simulink model "neighbour_and_local"  (R2020a)
settings: Solver=ode15s  StartTime=0.0  StopTime=200  FixedStep=1e-3
values from neighbouring files (symbols this model uses):
  A = A-B*Kctrl    [project2.m]
  Adj = tril(ones(6),-1) - tril(ones(6),-2)    [project2.m]
  B = [0; -9.9453]    [project2.m]
  c = ctemp*10    [project2.m]
  C = [708.27 0]    [project2.m]
  D = 0    [project2.m]
  Fl = -Fn    [project2.m]
  Fn = Pn*C'*inv(R)    [project2.m]
  K = inv(R)*B'*Pk    [project2.m]
  Pinning = zeros(6)    [project2.m]
  x0 = [0,0]    [project2.m]
  x1 = [0;1/707.27]    [project2.m]
settings Model: Creator=fmare  LastModifiedBy=fmare

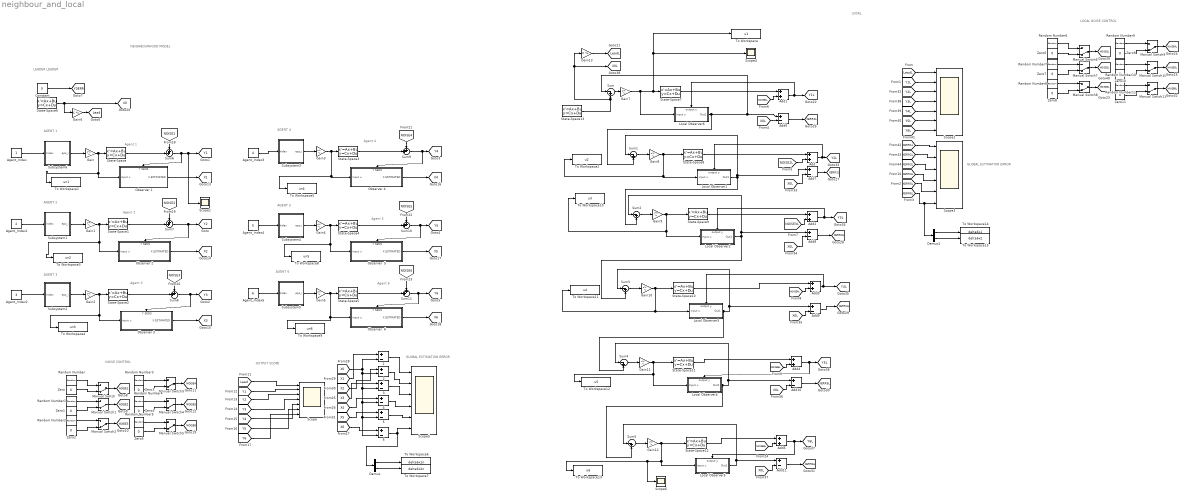
== system neighbour_and_local ==
  note: GLOBAL ESTIMATION ERROR
  note: AGENT 2
  note: NEIGHBOURHOOD MODEL
  note: OUTPUT SCOPE
  note: NOISE CONTROL
  note: Agent 6
  note: Agent 5
  note: Agent 4
  note: Agent 3
  note: Agent 1
  note: Agent 2
  note: AGENT 3
  note: AGENT 4
  note: AGENT 5
  note: AGENT 6
  note: AGENT 1
  note: LEADER
      | LEADER
  note: LOCAL NOISE CONTROL
  note: LOCAL
  note: GLOBAL ESTIMATION ERROR
  {1..6} (6 alike) : Sum  Inputs=+-
  Add{,1..5} (6 alike) : Sum
  Add{6..11} (6 alike) : Sum  Inputs=+-
  Agent_Index : Constant
  Agent_Index1 : Constant  Value=2
  Agent_Index2 : Constant  Value=3
  Agent_Index3 : Constant  Value=4
  Agent_Index4 : Constant  Value=5
  Agent_Index5 : Constant  Value=6
  Constant : Constant  Value=0
  Demux : Demux  Outputs=2
  Demux1 : Demux  Outputs=2
  Gain{,1..5,7..12} (12 alike) : Gain  Gain=c*K  Multiplication=Matrix(K*u)
  Gain13 : Gain  Gain=C  Multiplication=Matrix(K*u)
  Gain6 : Gain  Gain=C  Multiplication=Matrix(K*u)
  Local Observer1 : Subsystem
      settings: PortSchema="{\"entries\":[{\"content\":{\"sides\":[{\"content\":{\"connectorIds\":[\"In1\"]},\"type\":\"ConnectorPlacement.EquallySpacedRectSide\",\"uuid\":\"ce67de7f-91c0-4754-b336-8169ed1c06a3\"},{\"content\":{\"connectorIds\":[\"Out1\"],\"side\":\"RIGHT\"},\"type\":\"ConnectorPlacement.EquallySpacedRectSide\",\"uuid\":\"6e6b0d4a-9d22-40e2-b393-8f2d03ad4e6d\"},{\"content\":{\"connectorIds\":[\"In2\"],\"side\":\"TOP\"},\"type\":\"ConnectorPlacement.EquallySpacedRectSide\",\"uuid\":\"826e64ba-5ab3-47cb-8ff5-a35c256fda47\"}]},\"type\":\"ConnectorPlacement.EquallySpacedConnector\",\"uuid\":\"cb3a4a79-4d46-4198-893f-ba43cc9ed20a\"}],\"packageUris\":[\"http://schema.mathworks.com/mf0/Connector/19700101\"],\"version\":\"1.0\"}"
  Local Observer2 : Subsystem
      settings: ErrorFcn=x0(:,3)  PortSchema="{\"entries\":[{\"content\":{\"sides\":[{\"content\":{\"connectorIds\":[\"In1\"]},\"type\":\"ConnectorPlacement.EquallySpacedRectSide\",\"uuid\":\"ce67de7f-91c0-4754-b336-8169ed1c06a3\"},{\"content\":{\"connectorIds\":[\"Out1\"],\"side\":\"RIGHT\"},\"type\":\"ConnectorPlacement.EquallySpacedRectSide\",\"uuid\":\"6e6b0d4a-9d22-40e2-b393-8f2d03ad4e6d\"},{\"content\":{\"connectorIds\":[\"In2\"],\"side\":\"TOP\"},\"type\":\"ConnectorPlacement.EquallySpacedRectSide\",\"uuid\":\"826e64ba-5ab3-47cb-8ff5-a35c256fda47\"}]},\"type\":\"ConnectorPlacement.EquallySpacedConnector\",\"uuid\":\"cb3a4a79-4d46-4198-893f-ba43cc9ed20a\"}],\"packageUris\":[\"http://schema.mathworks.com/mf0/Connector/19700101\"],\"version\":\"1.0\"}"
  Local Observer3 : Subsystem
      settings: PortSchema="{\"entries\":[{\"content\":{\"sides\":[{\"content\":{\"connectorIds\":[\"In1\"]},\"type\":\"ConnectorPlacement.EquallySpacedRectSide\",\"uuid\":\"ce67de7f-91c0-4754-b336-8169ed1c06a3\"},{\"content\":{\"connectorIds\":[\"Out1\"],\"side\":\"RIGHT\"},\"type\":\"ConnectorPlacement.EquallySpacedRectSide\",\"uuid\":\"6e6b0d4a-9d22-40e2-b393-8f2d03ad4e6d\"},{\"content\":{\"connectorIds\":[\"In2\"],\"side\":\"TOP\"},\"type\":\"ConnectorPlacement.EquallySpacedRectSide\",\"uuid\":\"826e64ba-5ab3-47cb-8ff5-a35c256fda47\"}]},\"type\":\"ConnectorPlacement.EquallySpacedConnector\",\"uuid\":\"cb3a4a79-4d46-4198-893f-ba43cc9ed20a\"}],\"packageUris\":[\"http://schema.mathworks.com/mf0/Connector/19700101\"],\"version\":\"1.0\"}"
  Local Observer4 : Subsystem
      settings: PortSchema="{\"entries\":[{\"content\":{\"sides\":[{\"content\":{\"connectorIds\":[\"In1\"]},\"type\":\"ConnectorPlacement.EquallySpacedRectSide\",\"uuid\":\"ce67de7f-91c0-4754-b336-8169ed1c06a3\"},{\"content\":{\"connectorIds\":[\"Out1\"],\"side\":\"RIGHT\"},\"type\":\"ConnectorPlacement.EquallySpacedRectSide\",\"uuid\":\"6e6b0d4a-9d22-40e2-b393-8f2d03ad4e6d\"},{\"content\":{\"connectorIds\":[\"In2\"],\"side\":\"TOP\"},\"type\":\"ConnectorPlacement.EquallySpacedRectSide\",\"uuid\":\"826e64ba-5ab3-47cb-8ff5-a35c256fda47\"}]},\"type\":\"ConnectorPlacement.EquallySpacedConnector\",\"uuid\":\"cb3a4a79-4d46-4198-893f-ba43cc9ed20a\"}],\"packageUris\":[\"http://schema.mathworks.com/mf0/Connector/19700101\"],\"version\":\"1.0\"}"
  Local Observer5 : Subsystem
      settings: PortSchema="{\"entries\":[{\"content\":{\"sides\":[{\"content\":{\"connectorIds\":[\"In1\"]},\"type\":\"ConnectorPlacement.EquallySpacedRectSide\",\"uuid\":\"ce67de7f-91c0-4754-b336-8169ed1c06a3\"},{\"content\":{\"connectorIds\":[\"Out1\"],\"side\":\"RIGHT\"},\"type\":\"ConnectorPlacement.EquallySpacedRectSide\",\"uuid\":\"6e6b0d4a-9d22-40e2-b393-8f2d03ad4e6d\"},{\"content\":{\"connectorIds\":[\"In2\"],\"side\":\"TOP\"},\"type\":\"ConnectorPlacement.EquallySpacedRectSide\",\"uuid\":\"826e64ba-5ab3-47cb-8ff5-a35c256fda47\"}]},\"type\":\"ConnectorPlacement.EquallySpacedConnector\",\"uuid\":\"cb3a4a79-4d46-4198-893f-ba43cc9ed20a\"}],\"packageUris\":[\"http://schema.mathworks.com/mf0/Connector/19700101\"],\"version\":\"1.0\"}"
  Local Observer6 : Subsystem
      settings: PortSchema="{\"entries\":[{\"content\":{\"sides\":[{\"content\":{\"connectorIds\":[\"In1\"]},\"type\":\"ConnectorPlacement.EquallySpacedRectSide\",\"uuid\":\"ce67de7f-91c0-4754-b336-8169ed1c06a3\"},{\"content\":{\"connectorIds\":[\"Out1\"],\"side\":\"RIGHT\"},\"type\":\"ConnectorPlacement.EquallySpacedRectSide\",\"uuid\":\"6e6b0d4a-9d22-40e2-b393-8f2d03ad4e6d\"},{\"content\":{\"connectorIds\":[\"In2\"],\"side\":\"TOP\"},\"type\":\"ConnectorPlacement.EquallySpacedRectSide\",\"uuid\":\"826e64ba-5ab3-47cb-8ff5-a35c256fda47\"}]},\"type\":\"ConnectorPlacement.EquallySpacedConnector\",\"uuid\":\"cb3a4a79-4d46-4198-893f-ba43cc9ed20a\"}],\"packageUris\":[\"http://schema.mathworks.com/mf0/Connector/19700101\"],\"version\":\"1.0\"}"
  Manual Switch{,1..11} (12 alike) : ManualSwitch  CurrentSetting=0
  Observer  5 : Subsystem
      settings: PortSchema="{\"entries\":[{\"content\":{\"sides\":[{\"content\":{\"connectorIds\":[\"In1\"]},\"type\":\"ConnectorPlacement.EquallySpacedRectSide\",\"uuid\":\"b93c2c7e-291f-4b9d-8fda-1b2b099801ba\"},{\"content\":{\"connectorIds\":[\"Out1\"],\"side\":\"RIGHT\"},\"type\":\"ConnectorPlacement.EquallySpacedRectSide\",\"uuid\":\"bce36e82-6a20-4166-b86c-027f3aa24e2d\"},{\"content\":{\"connectorIds\":[\"In2\"],\"side\":\"TOP\"},\"type\":\"ConnectorPlacement.EquallySpacedRectSide\",\"uuid\":\"6cc367c2-dbc2-4b10-a825-48e36dcd66f7\"}]},\"type\":\"ConnectorPlacement.EquallySpacedConnector\",\"uuid\":\"fae6adff-b2a2-4da1-a9d8-7a0ab3ce0116\"}],\"packageUris\":[\"http://schema.mathworks.com/mf0/Connector/R2020b\"],\"version\":\"1.0\"}"
  Observer  6 : Subsystem
      settings: PortSchema="{\"entries\":[{\"content\":{\"sides\":[{\"content\":{\"connectorIds\":[\"In1\"]},\"type\":\"ConnectorPlacement.EquallySpacedRectSide\",\"uuid\":\"b93c2c7e-291f-4b9d-8fda-1b2b099801ba\"},{\"content\":{\"connectorIds\":[\"Out1\"],\"side\":\"RIGHT\"},\"type\":\"ConnectorPlacement.EquallySpacedRectSide\",\"uuid\":\"bce36e82-6a20-4166-b86c-027f3aa24e2d\"},{\"content\":{\"connectorIds\":[\"In2\"],\"side\":\"TOP\"},\"type\":\"ConnectorPlacement.EquallySpacedRectSide\",\"uuid\":\"6cc367c2-dbc2-4b10-a825-48e36dcd66f7\"}]},\"type\":\"ConnectorPlacement.EquallySpacedConnector\",\"uuid\":\"fae6adff-b2a2-4da1-a9d8-7a0ab3ce0116\"}],\"packageUris\":[\"http://schema.mathworks.com/mf0/Connector/R2020b\"],\"version\":\"1.0\"}"
  Observer 1 : Subsystem
      settings: PortSchema="{\"entries\":[{\"content\":{\"sides\":[{\"content\":{\"connectorIds\":[\"In1\"]},\"type\":\"ConnectorPlacement.EquallySpacedRectSide\",\"uuid\":\"b93c2c7e-291f-4b9d-8fda-1b2b099801ba\"},{\"content\":{\"connectorIds\":[\"Out1\"],\"side\":\"RIGHT\"},\"type\":\"ConnectorPlacement.EquallySpacedRectSide\",\"uuid\":\"bce36e82-6a20-4166-b86c-027f3aa24e2d\"},{\"content\":{\"connectorIds\":[\"In2\"],\"side\":\"TOP\"},\"type\":\"ConnectorPlacement.EquallySpacedRectSide\",\"uuid\":\"6cc367c2-dbc2-4b10-a825-48e36dcd66f7\"}]},\"type\":\"ConnectorPlacement.EquallySpacedConnector\",\"uuid\":\"fae6adff-b2a2-4da1-a9d8-7a0ab3ce0116\"}],\"packageUris\":[\"http://schema.mathworks.com/mf0/Connector/R2020b\"],\"version\":\"1.0\"}"
  Observer 2 : Subsystem
      settings: PortSchema="{\"entries\":[{\"content\":{\"sides\":[{\"content\":{\"connectorIds\":[\"In1\"]},\"type\":\"ConnectorPlacement.EquallySpacedRectSide\",\"uuid\":\"b93c2c7e-291f-4b9d-8fda-1b2b099801ba\"},{\"content\":{\"connectorIds\":[\"Out1\"],\"side\":\"RIGHT\"},\"type\":\"ConnectorPlacement.EquallySpacedRectSide\",\"uuid\":\"bce36e82-6a20-4166-b86c-027f3aa24e2d\"},{\"content\":{\"connectorIds\":[\"In2\"],\"side\":\"TOP\"},\"type\":\"ConnectorPlacement.EquallySpacedRectSide\",\"uuid\":\"6cc367c2-dbc2-4b10-a825-48e36dcd66f7\"}]},\"type\":\"ConnectorPlacement.EquallySpacedConnector\",\"uuid\":\"fae6adff-b2a2-4da1-a9d8-7a0ab3ce0116\"}],\"packageUris\":[\"http://schema.mathworks.com/mf0/Connector/R2020b\"],\"version\":\"1.0\"}"
  Observer 3 : Subsystem
      settings: PortSchema="{\"entries\":[{\"content\":{\"sides\":[{\"content\":{\"connectorIds\":[\"In1\"]},\"type\":\"ConnectorPlacement.EquallySpacedRectSide\",\"uuid\":\"b93c2c7e-291f-4b9d-8fda-1b2b099801ba\"},{\"content\":{\"connectorIds\":[\"Out1\"],\"side\":\"RIGHT\"},\"type\":\"ConnectorPlacement.EquallySpacedRectSide\",\"uuid\":\"bce36e82-6a20-4166-b86c-027f3aa24e2d\"},{\"content\":{\"connectorIds\":[\"In2\"],\"side\":\"TOP\"},\"type\":\"ConnectorPlacement.EquallySpacedRectSide\",\"uuid\":\"6cc367c2-dbc2-4b10-a825-48e36dcd66f7\"}]},\"type\":\"ConnectorPlacement.EquallySpacedConnector\",\"uuid\":\"fae6adff-b2a2-4da1-a9d8-7a0ab3ce0116\"}],\"packageUris\":[\"http://schema.mathworks.com/mf0/Connector/R2020b\"],\"version\":\"1.0\"}"
  Observer 4 : Subsystem
      settings: PortSchema="{\"entries\":[{\"content\":{\"sides\":[{\"content\":{\"connectorIds\":[\"In1\"]},\"type\":\"ConnectorPlacement.EquallySpacedRectSide\",\"uuid\":\"b93c2c7e-291f-4b9d-8fda-1b2b099801ba\"},{\"content\":{\"connectorIds\":[\"Out1\"],\"side\":\"RIGHT\"},\"type\":\"ConnectorPlacement.EquallySpacedRectSide\",\"uuid\":\"bce36e82-6a20-4166-b86c-027f3aa24e2d\"},{\"content\":{\"connectorIds\":[\"In2\"],\"side\":\"TOP\"},\"type\":\"ConnectorPlacement.EquallySpacedRectSide\",\"uuid\":\"6cc367c2-dbc2-4b10-a825-48e36dcd66f7\"}]},\"type\":\"ConnectorPlacement.EquallySpacedConnector\",\"uuid\":\"fae6adff-b2a2-4da1-a9d8-7a0ab3ce0116\"}],\"packageUris\":[\"http://schema.mathworks.com/mf0/Connector/R2020b\"],\"version\":\"1.0\"}"
  Random Number{,1..5} (6 alike) : RandomNumber  Variance=0.5  SampleTime=0.1
  Random Number{6..11} (6 alike) : RandomNumber  SampleTime=0.1
  Scope : Scope  NumInputPorts=7
  Scope1 : Scope
  Scope2 : Scope  NumInputPorts=7
  Scope3 : Scope  NumInputPorts=6
  Scope4 : Scope
  Scope5 : Scope  NumInputPorts=6
  Scope6 : Scope
  State-Space : StateSpace  A=A  B=B  C=C  D=D  InitialCondition=x0(:,1)
  State-Space1 : StateSpace  A=A  B=B  C=C  D=D  InitialCondition=x0(:,2)
  State-Space10 : StateSpace  A=A  B=B  C=C  D=D  InitialCondition=x0(:,4)
  State-Space11 : StateSpace  A=A  B=B  C=C  D=D  InitialCondition=x0(:,5)
  State-Space12 : StateSpace  A=A  B=B  C=C  D=D  InitialCondition=x0(:,6)
  State-Space13 : StateSpace  A=A  B=B  C=eye(2)  D=zeros(2,1)  InitialCondition=x1
  State-Space2 : StateSpace  A=A  B=B  C=C  D=D  InitialCondition=x0(:,3)
  State-Space3 : StateSpace  A=A  B=B  C=C  D=D  InitialCondition=x0(:,4)
  State-Space4 : StateSpace  A=A  B=B  C=C  D=D  InitialCondition=x0(:,5)
  State-Space5 : StateSpace  A=A  B=B  C=C  D=D  InitialCondition=x0(:,6)
  State-Space6 : StateSpace  A=A  B=B  C=eye(2)  D=zeros(2,1)  InitialCondition=x1
  State-Space7 : StateSpace  A=A  B=B  C=C  D=D  InitialCondition=x0(:,1)
  State-Space8 : StateSpace  A=A  B=B  C=C  D=D  InitialCondition=x0(:,2)
  State-Space9 : StateSpace  A=A  B=B  C=C  D=D  InitialCondition=x0(:,3)
  Subsystem1 : Subsystem
  Subsystem2 : Subsystem
  Subsystem3 : Subsystem
  Subsystem4 : Subsystem
  Subsystem5 : Subsystem
  Subsystem6 : Subsystem
  Sum{,1..5} (6 alike) : Sum  Inputs=|-+
  Sum{6..11} (6 alike) : Sum  Inputs=++|
  To Workspace : ToWorkspace  VariableName=u1  SaveFormat=Timeseries  SampleTime=-1
      settings: Save2DSignal=2-D array (concatenate along first dimension)
  To Workspace1 : ToWorkspace  VariableName=un1  SaveFormat=Timeseries  SampleTime=-1
      settings: Save2DSignal=2-D array (concatenate along first dimension)
  To Workspace10 : ToWorkspace  VariableName=u3  SaveFormat=Timeseries  SampleTime=-1
      settings: Save2DSignal=2-D array (concatenate along first dimension)
  To Workspace11 : ToWorkspace  VariableName=u4  SaveFormat=Timeseries  SampleTime=-1
      settings: Save2DSignal=2-D array (concatenate along first dimension)
  To Workspace12 : ToWorkspace  VariableName=u5  SaveFormat=Timeseries  SampleTime=-1
      settings: Save2DSignal=2-D array (concatenate along first dimension)
  To Workspace13 : ToWorkspace  VariableName=u6  SaveFormat=Timeseries  SampleTime=-1
      settings: Save2DSignal=2-D array (concatenate along first dimension)
  To Workspace14 : ToWorkspace  VariableName=delta6x1  SaveFormat=Timeseries  SampleTime=-1
      settings: Save2DSignal=2-D array (concatenate along first dimension)
  To Workspace15 : ToWorkspace  VariableName=delta6x2  SaveFormat=Timeseries  SampleTime=-1
      settings: Save2DSignal=2-D array (concatenate along first dimension)
  To Workspace2 : ToWorkspace  VariableName=u2  SaveFormat=Timeseries  SampleTime=-1
      settings: Save2DSignal=2-D array (concatenate along first dimension)
  To Workspace3 : ToWorkspace  VariableName=un2  SaveFormat=Timeseries  SampleTime=-1
      settings: Save2DSignal=2-D array (concatenate along first dimension)
  To Workspace4 : ToWorkspace  VariableName=un3  SaveFormat=Timeseries  SampleTime=-1
      settings: Save2DSignal=2-D array (concatenate along first dimension)
  To Workspace5 : ToWorkspace  VariableName=un4  SaveFormat=Timeseries  SampleTime=-1
      settings: Save2DSignal=2-D array (concatenate along first dimension)
  To Workspace6 : ToWorkspace  VariableName=delta6x1n  SaveFormat=Timeseries  SampleTime=-1
      settings: Save2DSignal=2-D array (concatenate along first dimension)
  To Workspace7 : ToWorkspace  VariableName=delta6x2n  SaveFormat=Timeseries  SampleTime=-1
      settings: Save2DSignal=2-D array (concatenate along first dimension)
  To Workspace8 : ToWorkspace  VariableName=un5  SaveFormat=Timeseries  SampleTime=-1
      settings: Save2DSignal=2-D array (concatenate along first dimension)
  To Workspace9 : ToWorkspace  VariableName=un6  SaveFormat=Timeseries  SampleTime=-1
      settings: Save2DSignal=2-D array (concatenate along first dimension)
  Zero{,1..11} (12 alike) : Constant  Value=0  OutDataTypeStr=Inherit: Inherit via back propagation
  tag scope: Lead=global, LeadL=global, NOISE1=global, NOISE1L=global, NOISE2=global, NOISE2L=global, NOISE3=global, NOISE3L=global, NOISE4=global, NOISE4L=global, NOISE5=global, NOISE5L=global, NOISE6=global, NOISE6L=global, X0=global, X0L=global, X1=global, X2=global, X3=global, X4=global, X5=global, X6=global, XERR1L=global, XERR2L=global, XERR3L=global, XERR4L=global, XERR5L=global, XERR6L=global, Y0ERR=global, Y1=global, Y1L=global, Y2=global, Y2L=global, Y3=global, Y3L=global, Y4=global, Y4L=global, Y5=global, Y5L=global, Y6=global, Y6L=global
  wires:
  State-Space3/1 -> Sum9/2
  State-Space4/1 -> Sum10/2
  State-Space6/1 -> [X0], Gain6/1
  State-Space5/1 -> Sum11/2
  State-Space/1 -> Sum6/2
  Gain2/1 -> To Workspace4/1, Observer 3/1(input u), State-Space2/1
  Gain1/1 -> To Workspace3/1, Observer 2/1(input u), State-Space1/1
  Gain5/1 -> State-Space5/1, To Workspace9/1, Observer  6/1(input u)
  State-Space2/1 -> Sum8/2
  Gain/1 -> To Workspace1/1, Observer 1/1(input u), State-Space/1
  State-Space1/1 -> Sum7/2
  Gain3/1 -> State-Space3/1, To Workspace5/1, Observer 4/1(input u)
  Observer 1/1(X ESTIMATED) -> [X1]
  Observer 2/1(X ESTIMATED) -> [X2]
  Observer 3/1(X ESTIMATED) -> [X3]
  Observer 4/1(X ESTIMATED) -> [X4]
  Observer  5/1(X ESTIMATED) -> [X5]
  Observer  6/1(X ESTIMATED) -> [X6]
  [Lead] -> Scope/1
  [Y1] -> Scope/2
  [Y2] -> Scope/3
  [Y3] -> Scope/4
  [Y4] -> Scope/5
  [Y5] -> Scope/6
  [Y6] -> Scope/7
  Gain6/1 -> [Lead]
  Constant/1 -> [Y0ERR]
  Sum6/1 -> Scope1/1, [Y1], Observer 1/2(Y SENS)
  Sum10/1 -> [Y5], Observer  5/2(Y SENS)
  Sum9/1 -> [Y4], Observer 4/2(Y SENS)
  Sum8/1 -> [Y3], Observer 3/2(Y SENS)
  Sum7/1 -> [Y2], Observer 2/2(Y SENS)
  [NOISE2] -> Sum7/1
  [NOISE1] -> Sum6/1
  [NOISE3] -> Sum8/1
  [NOISE4] -> Sum9/1
  [NOISE5] -> Sum10/1
  [NOISE6] -> Sum11/1
  Manual Switch/1 -> [NOISE1]
  Random Number/1 -> Manual Switch/1
  Zero/1 -> Manual Switch/2
  Random Number1/1 -> Manual Switch1/1
  Manual Switch1/1 -> [NOISE2]
  Zero1/1 -> Manual Switch1/2
  Random Number2/1 -> Manual Switch2/1
  Manual Switch2/1 -> [NOISE3]
  Zero2/1 -> Manual Switch2/2
  Random Number3/1 -> Manual Switch3/1
  Manual Switch3/1 -> [NOISE4]
  Zero3/1 -> Manual Switch3/2
  Random Number4/1 -> Manual Switch4/1
  Manual Switch4/1 -> [NOISE5]
  Zero4/1 -> Manual Switch4/2
  Random Number5/1 -> Manual Switch5/1
  Manual Switch5/1 -> [NOISE6]
  Zero5/1 -> Manual Switch5/2
  Subsystem6/1(eps_i) -> Gain/1
  Subsystem1/1(eps_i) -> Gain1/1
  Agent_Index2/1 -> Subsystem2/1(Index)
  Subsystem2/1(eps_i) -> Gain2/1
  Agent_Index3/1 -> Subsystem3/1(Index)
  Subsystem3/1(eps_i) -> Gain3/1
  Agent_Index4/1 -> Subsystem4/1(Index)
  Subsystem4/1(eps_i) -> Gain4/1
  Agent_Index5/1 -> Subsystem5/1(Index)
  Subsystem5/1(eps_i) -> Gain5/1
  [X0] -> 6/2, 5/2, 4/2, 3/2, 2/2, 1/2
  [X4] -> 4/1
  5/1 -> Scope5/5
  1/1 -> Scope5/1
  4/1 -> Scope5/4
  [X1] -> 1/1
  Demux/1 -> To Workspace6/1
  [X6] -> 6/1
  Demux/2 -> To Workspace7/1
  [X2] -> 2/1
  2/1 -> Scope5/2
  6/1 -> Demux/1, Scope5/6
  [X5] -> 5/1
  [X3] -> 3/1
  3/1 -> Scope5/3
  Agent_Index1/1 -> Subsystem1/1(Index)
  Agent_Index/1 -> Subsystem6/1(Index)
  Gain4/1 -> State-Space4/1, To Workspace8/1, Observer  5/1(input u)
  Add9/1 -> [XERR4L]
  Local Observer3/1(Out1) -> Sum3/1, Add9/1, Sum4/2
  Add5/1 -> Local Observer5/2(output y), [Y6L]
  Demux1/2 -> To Workspace15/1
  State-Space9/1 -> Add2/1
  Zero10/1 -> Manual Switch10/2
  Zero9/1 -> Manual Switch9/2
  Zero8/1 -> Manual Switch8/2
  Manual Switch8/1 -> [NOISE3L]
  Manual Switch10/1 -> [NOISE5L]
  Random Number9/1 -> Manual Switch9/1
  Gain13/1 -> [LeadL]
  Random Number6/1 -> Manual Switch6/1
  [XERR6L] -> Demux1/1, Scope3/6
  Add/1 -> Local Observer1/2(output y), [Y2L]
  [Y3L] -> Scope2/4
  [XERR4L] -> Scope3/4
  [Y6L] -> Scope2/7
  [Y2L] -> Scope2/3
  [Y1L] -> Scope2/2
  [LeadL] -> Scope2/1
  Gain9/1 -> Local Observer2/1(input u), To Workspace10/1, State-Space9/1
  [X0L] -> Add8/2
  Local Observer5/1(Out1) -> Add11/1, Sum5/1
  Add11/1 -> [XERR6L]
  [NOISE1L] -> Add1/2
  [XERR1L] -> Scope3/1
  [NOISE2L] -> Add/2
  Sum1/1 -> Gain8/1
  Zero6/1 -> Manual Switch6/2
  Add6/1 -> [XERR1L]
  State-Space12/1 -> Add5/1
  Zero7/1 -> Manual Switch7/2
  [X0L] -> Add11/2
  Add1/1 -> Local Observer6/2(output y), [Y1L]
  Gain12/1 -> Local Observer5/1(input u), Scope6/1, To Workspace13/1, State-Space12/1
  State-Space7/1 -> Add1/1
  Add2/1 -> [Y3L], Local Observer2/2(output y)
  State-Space13/1 -> Sum/2, [X0L], Gain13/1
  Sum3/1 -> Gain10/1
  Sum4/1 -> Gain11/1
  Sum2/1 -> Gain9/1
  Gain8/1 -> To Workspace2/1, Local Observer1/1(input u), State-Space8/1
  Add8/1 -> [XERR3L]
  [XERR5L] -> Scope3/5
  Add7/1 -> [XERR2L]
  State-Space8/1 -> Add/1
  Manual Switch6/1 -> [NOISE1L]
  [NOISE5L] -> Add4/2
  Random Number10/1 -> Manual Switch10/1
  [NOISE3L] -> Add2/2
  Zero11/1 -> Manual Switch11/2
  State-Space10/1 -> Add3/1
  [NOISE4L] -> Add3/2
  Random Number7/1 -> Manual Switch7/1
  Gain11/1 -> Local Observer4/1(input u), To Workspace12/1, State-Space11/1
  Local Observer6/1(Out1) -> Sum/1, Add6/1, Sum1/2
  [X0L] -> Add6/2
  Local Observer2/1(Out1) -> Sum2/1, Add8/1, Sum3/2
  Sum5/1 -> Gain12/1
  [Y5L] -> Scope2/6
  Local Observer1/1(Out1) -> Sum1/1, Add7/1, Sum2/2
  Demux1/1 -> To Workspace14/1
  Add3/1 -> Local Observer3/2(output y), [Y4L]
  [X0L] -> Add7/2
  State-Space11/1 -> Add4/1
  [XERR2L] -> Scope3/2
  Sum/1 -> Gain7/1
  [X0L] -> Add10/2
  Gain10/1 -> To Workspace11/1, Local Observer3/1(input u), State-Space10/1
  Random Number11/1 -> Manual Switch11/1
  Random Number8/1 -> Manual Switch8/1
  Gain7/1 -> Local Observer6/1(input u), To Workspace/1, Scope4/1, State-Space7/1
  Add4/1 -> [Y5L], Local Observer4/2(output y)
  [Y4L] -> Scope2/5
  Local Observer4/1(Out1) -> Add10/1, Sum4/1, Sum5/2
  [X0L] -> Add9/2
  Add10/1 -> [XERR5L]
  Manual Switch7/1 -> [NOISE2L]
  [NOISE6L] -> Add5/2
  Manual Switch11/1 -> [NOISE6L]
  Manual Switch9/1 -> [NOISE4L]
  [XERR3L] -> Scope3/3
  Sum11/1 -> [Y6], Observer  6/2(Y SENS)

== system neighbour_and_local/Local Observer1 ==
  note: x estimated
  note: xdot
  input u : Inport
  output y : Inport  Port=2
  Add : Sum  Inputs=++-
  Gain : Gain  Gain=B  Multiplication=Matrix(K*u)
  Gain1 : Gain  Gain=c*Fl  Multiplication=Matrix(K*u)
  Gain2 : Gain  Gain=C  Multiplication=Matrix(K*u)
  Integrator : Integrator  InitialCondition=x0(:,2)
  State estimation : Gain  Gain=A  Multiplication=Matrix(K*u)
  Subtract : Sum  Inputs=+-
  Out1 : Outport  PortDimensions=[2,1]
  wires:
  input u/1 -> Gain/1
  output y/1 -> Subtract/1
  Gain/1 -> Add/2
  Gain1/1 -> Add/3
  Add/1 -> Integrator/1
  State estimation/1 -> Add/1
  Integrator/1 -> Out1/1, State estimation/1, Gain2/1
  Gain2/1 -> Subtract/2
  Subtract/1 -> Gain1/1

== system neighbour_and_local/Local Observer2 ==
  note: x estimated
  note: xdot
  input u : Inport
  output y : Inport  Port=2
  Add : Sum  Inputs=++-
  Gain : Gain  Gain=B  Multiplication=Matrix(K*u)
  Gain1 : Gain  Gain=c*Fl  Multiplication=Matrix(K*u)
  Gain2 : Gain  Gain=C  Multiplication=Matrix(K*u)
  Integrator : Integrator  InitialCondition=x0(:,3)
  State estimation : Gain  Gain=A  Multiplication=Matrix(K*u)
  Subtract : Sum  Inputs=+-
  Out1 : Outport  PortDimensions=[2,1]
  wires:
  input u/1 -> Gain/1
  output y/1 -> Subtract/1
  Gain/1 -> Add/2
  Gain1/1 -> Add/3
  Add/1 -> Integrator/1
  State estimation/1 -> Add/1
  Integrator/1 -> Out1/1, State estimation/1, Gain2/1
  Gain2/1 -> Subtract/2
  Subtract/1 -> Gain1/1

== system neighbour_and_local/Local Observer3 ==
  note: x estimated
  note: xdot
  input u : Inport
  output y : Inport  Port=2
  Add : Sum  Inputs=++-
  Gain : Gain  Gain=B  Multiplication=Matrix(K*u)
  Gain1 : Gain  Gain=c*Fl  Multiplication=Matrix(K*u)
  Gain2 : Gain  Gain=C  Multiplication=Matrix(K*u)
  Integrator : Integrator  InitialCondition=x0(:,4)
  State estimation : Gain  Gain=A  Multiplication=Matrix(K*u)
  Subtract : Sum  Inputs=+-
  Out1 : Outport  PortDimensions=[2,1]
  wires:
  input u/1 -> Gain/1
  output y/1 -> Subtract/1
  Gain/1 -> Add/2
  Gain1/1 -> Add/3
  Add/1 -> Integrator/1
  State estimation/1 -> Add/1
  Integrator/1 -> Out1/1, State estimation/1, Gain2/1
  Gain2/1 -> Subtract/2
  Subtract/1 -> Gain1/1

== system neighbour_and_local/Local Observer4 ==
  note: x estimated
  note: xdot
  input u : Inport
  output y : Inport  Port=2
  Add : Sum  Inputs=++-
  Gain : Gain  Gain=B  Multiplication=Matrix(K*u)
  Gain1 : Gain  Gain=c*Fl  Multiplication=Matrix(K*u)
  Gain2 : Gain  Gain=C  Multiplication=Matrix(K*u)
  Integrator : Integrator  InitialCondition=x0(:,5)
  State estimation : Gain  Gain=A  Multiplication=Matrix(K*u)
  Subtract : Sum  Inputs=+-
  Out1 : Outport  PortDimensions=[2,1]
  wires:
  input u/1 -> Gain/1
  output y/1 -> Subtract/1
  Gain/1 -> Add/2
  Gain1/1 -> Add/3
  Add/1 -> Integrator/1
  State estimation/1 -> Add/1
  Integrator/1 -> Out1/1, State estimation/1, Gain2/1
  Gain2/1 -> Subtract/2
  Subtract/1 -> Gain1/1

== system neighbour_and_local/Local Observer5 ==
  note: x estimated
  note: xdot
  input u : Inport
  output y : Inport  Port=2
  Add : Sum  Inputs=++-
  Gain : Gain  Gain=B  Multiplication=Matrix(K*u)
  Gain1 : Gain  Gain=c*Fl  Multiplication=Matrix(K*u)
  Gain2 : Gain  Gain=C  Multiplication=Matrix(K*u)
  Integrator : Integrator  InitialCondition=x0(:,6)
  State estimation : Gain  Gain=A  Multiplication=Matrix(K*u)
  Subtract : Sum  Inputs=+-
  Out1 : Outport  PortDimensions=[2,1]
  wires:
  input u/1 -> Gain/1
  output y/1 -> Subtract/1
  Gain/1 -> Add/2
  Gain1/1 -> Add/3
  Add/1 -> Integrator/1
  State estimation/1 -> Add/1
  Integrator/1 -> Out1/1, State estimation/1, Gain2/1
  Gain2/1 -> Subtract/2
  Subtract/1 -> Gain1/1

== system neighbour_and_local/Local Observer6 ==
  note: x estimated
  note: xdot
  input u : Inport
  output y : Inport  Port=2
  Add : Sum  Inputs=++-
  Gain : Gain  Gain=B  Multiplication=Matrix(K*u)
  Gain1 : Gain  Gain=c*Fl  Multiplication=Matrix(K*u)
  Gain2 : Gain  Gain=C  Multiplication=Matrix(K*u)
  Integrator : Integrator  InitialCondition=x0(:,1)
  State estimation : Gain  Gain=A  Multiplication=Matrix(K*u)
  Subtract : Sum  Inputs=+-
  Out1 : Outport  PortDimensions=[2,1]
  wires:
  input u/1 -> Gain/1
  output y/1 -> Subtract/1
  Gain/1 -> Add/2
  Gain1/1 -> Add/3
  Add/1 -> Integrator/1
  State estimation/1 -> Add/1
  Integrator/1 -> Out1/1, State estimation/1, Gain2/1
  Subtract/1 -> Gain1/1
  Gain2/1 -> Subtract/2

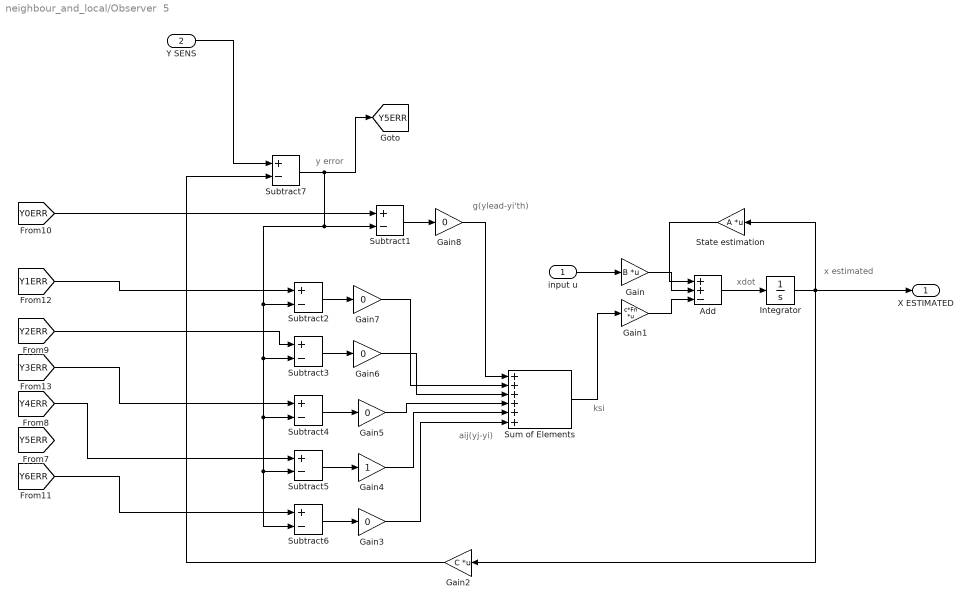
== system neighbour_and_local/Observer  5 ==
  note: aij(yj-yi)
  note: g(ylead-yi'th)
  note: ksi
  note: y error
  note: x estimated
  note: xdot
  input u : Inport
  Y SENS : Inport  Port=2
  Add : Sum  Inputs=++-
  Gain : Gain  Gain=B  Multiplication=Matrix(K*u)
  Gain1 : Gain  Gain=c*Fn  Multiplication=Matrix(K*u)
  Gain2 : Gain  Gain=C  Multiplication=Matrix(K*u)
  Gain{3,5..8} (5 alike) : Gain  Gain=0
  Gain4 : Gain
  Integrator : Integrator  InitialCondition=x0(:,5)
  State estimation : Gain  Gain=A  Multiplication=Matrix(K*u)
  Subtract{1..7} (7 alike) : Sum  Inputs=+-
  Sum of Elements : Sum  Inputs=++++++
  X ESTIMATED : Outport
  tag scope: Y5ERR=global
  wires:
  input u/1 -> Gain/1
  [Y0ERR] -> Subtract1/1
  Gain/1 -> Add/2
  Gain1/1 -> Add/3
  Add/1 -> Integrator/1
  State estimation/1 -> Add/1
  Integrator/1 -> X ESTIMATED/1, Gain2/1, State estimation/1
  Sum of Elements/1 -> Gain1/1
  Gain2/1 -> Subtract7/2
  [Y1ERR] -> Subtract2/1
  [Y2ERR] -> Subtract3/1
  [Y3ERR] -> Subtract4/1
  [Y4ERR] -> Subtract5/1
  [Y6ERR] -> Subtract6/1
  Subtract2/1 -> Gain7/1
  Subtract3/1 -> Gain6/1
  Subtract4/1 -> Gain5/1
  Subtract5/1 -> Gain4/1
  Subtract6/1 -> Gain3/1
  Subtract1/1 -> Gain8/1
  Gain8/1 -> Sum of Elements/1
  Gain7/1 -> Sum of Elements/2
  Gain6/1 -> Sum of Elements/3
  Gain3/1 -> Sum of Elements/6
  Gain5/1 -> Sum of Elements/4
  Gain4/1 -> Sum of Elements/5
  Subtract7/1 -> [Y5ERR], Subtract2/2, Subtract3/2, Subtract4/2, Subtract5/2, Subtract6/2, Subtract1/2
  Y SENS/1 -> Subtract7/1

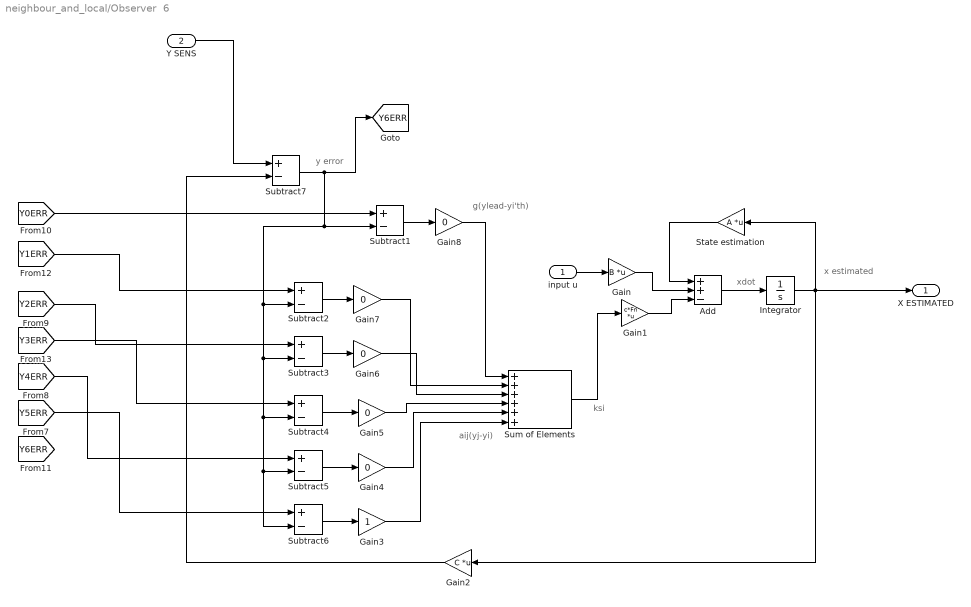
== system neighbour_and_local/Observer  6 ==
  note: aij(yj-yi)
  note: g(ylead-yi'th)
  note: ksi
  note: y error
  note: x estimated
  note: xdot
  input u : Inport
  Y SENS : Inport  Port=2
  Add : Sum  Inputs=++-
  Gain : Gain  Gain=B  Multiplication=Matrix(K*u)
  Gain1 : Gain  Gain=c*Fn  Multiplication=Matrix(K*u)
  Gain2 : Gain  Gain=C  Multiplication=Matrix(K*u)
  Gain3 : Gain
  Gain{4..8} (5 alike) : Gain  Gain=0
  Integrator : Integrator  InitialCondition=x0(:,6)
  State estimation : Gain  Gain=A  Multiplication=Matrix(K*u)
  Subtract{1..7} (7 alike) : Sum  Inputs=+-
  Sum of Elements : Sum  Inputs=++++++
  X ESTIMATED : Outport
  tag scope: Y6ERR=global
  wires:
  input u/1 -> Gain/1
  [Y0ERR] -> Subtract1/1
  Gain/1 -> Add/2
  Gain1/1 -> Add/3
  Add/1 -> Integrator/1
  State estimation/1 -> Add/1
  Integrator/1 -> X ESTIMATED/1, Gain2/1, State estimation/1
  Sum of Elements/1 -> Gain1/1
  Gain2/1 -> Subtract7/2
  [Y1ERR] -> Subtract2/1
  [Y2ERR] -> Subtract3/1
  [Y3ERR] -> Subtract4/1
  [Y4ERR] -> Subtract5/1
  [Y5ERR] -> Subtract6/1
  Subtract2/1 -> Gain7/1
  Subtract3/1 -> Gain6/1
  Subtract4/1 -> Gain5/1
  Subtract5/1 -> Gain4/1
  Subtract6/1 -> Gain3/1
  Subtract1/1 -> Gain8/1
  Gain8/1 -> Sum of Elements/1
  Gain7/1 -> Sum of Elements/2
  Gain6/1 -> Sum of Elements/3
  Gain3/1 -> Sum of Elements/6
  Gain5/1 -> Sum of Elements/4
  Gain4/1 -> Sum of Elements/5
  Subtract7/1 -> [Y6ERR], Subtract2/2, Subtract3/2, Subtract4/2, Subtract5/2, Subtract6/2, Subtract1/2
  Y SENS/1 -> Subtract7/1

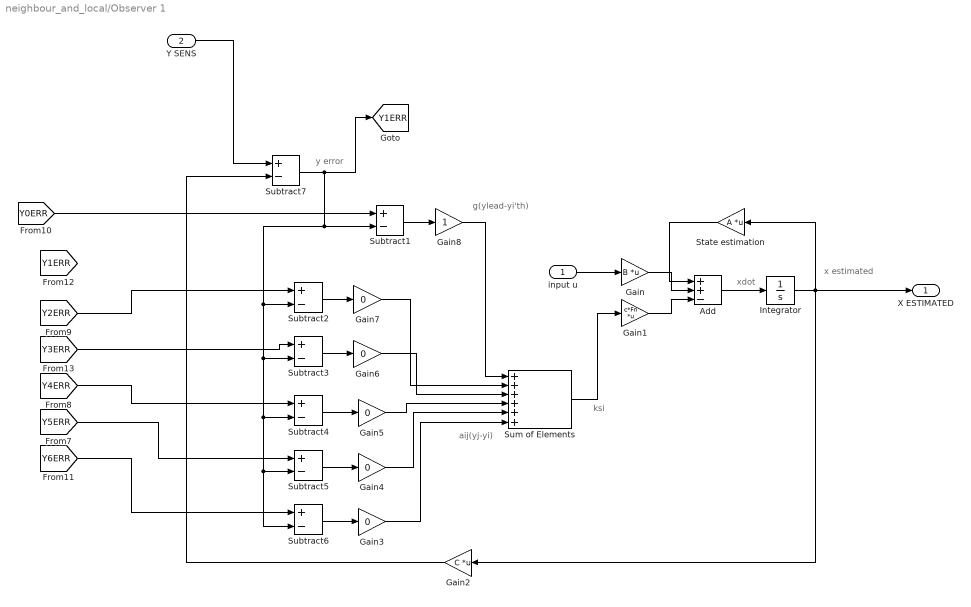
== system neighbour_and_local/Observer 1 ==
  note: aij(yj-yi)
  note: g(ylead-yi'th)
  note: ksi
  note: y error
  note: x estimated
  note: xdot
  input u : Inport
  Y SENS : Inport  Port=2
  Add : Sum  Inputs=++-
  Gain : Gain  Gain=B  Multiplication=Matrix(K*u)
  Gain1 : Gain  Gain=c*Fn  Multiplication=Matrix(K*u)
  Gain2 : Gain  Gain=C  Multiplication=Matrix(K*u)
  Gain{3..7} (5 alike) : Gain  Gain=0
  Gain8 : Gain
  Integrator : Integrator  InitialCondition=x0(:,1)
  State estimation : Gain  Gain=A  Multiplication=Matrix(K*u)
  Subtract{1..7} (7 alike) : Sum  Inputs=+-
  Sum of Elements : Sum  Inputs=++++++
  X ESTIMATED : Outport
  tag scope: Y1ERR=global
  wires:
  input u/1 -> Gain/1
  [Y0ERR] -> Subtract1/1
  Gain/1 -> Add/2
  Gain1/1 -> Add/3
  Add/1 -> Integrator/1
  State estimation/1 -> Add/1
  Integrator/1 -> X ESTIMATED/1, Gain2/1, State estimation/1
  Sum of Elements/1 -> Gain1/1
  Gain2/1 -> Subtract7/2
  [Y2ERR] -> Subtract2/1
  [Y3ERR] -> Subtract3/1
  [Y4ERR] -> Subtract4/1
  [Y5ERR] -> Subtract5/1
  [Y6ERR] -> Subtract6/1
  Subtract2/1 -> Gain7/1
  Subtract3/1 -> Gain6/1
  Subtract4/1 -> Gain5/1
  Subtract5/1 -> Gain4/1
  Subtract6/1 -> Gain3/1
  Subtract1/1 -> Gain8/1
  Gain8/1 -> Sum of Elements/1
  Gain7/1 -> Sum of Elements/2
  Gain6/1 -> Sum of Elements/3
  Gain3/1 -> Sum of Elements/6
  Gain5/1 -> Sum of Elements/4
  Gain4/1 -> Sum of Elements/5
  Subtract7/1 -> [Y1ERR], Subtract2/2, Subtract3/2, Subtract4/2, Subtract5/2, Subtract6/2, Subtract1/2
  Y SENS/1 -> Subtract7/1

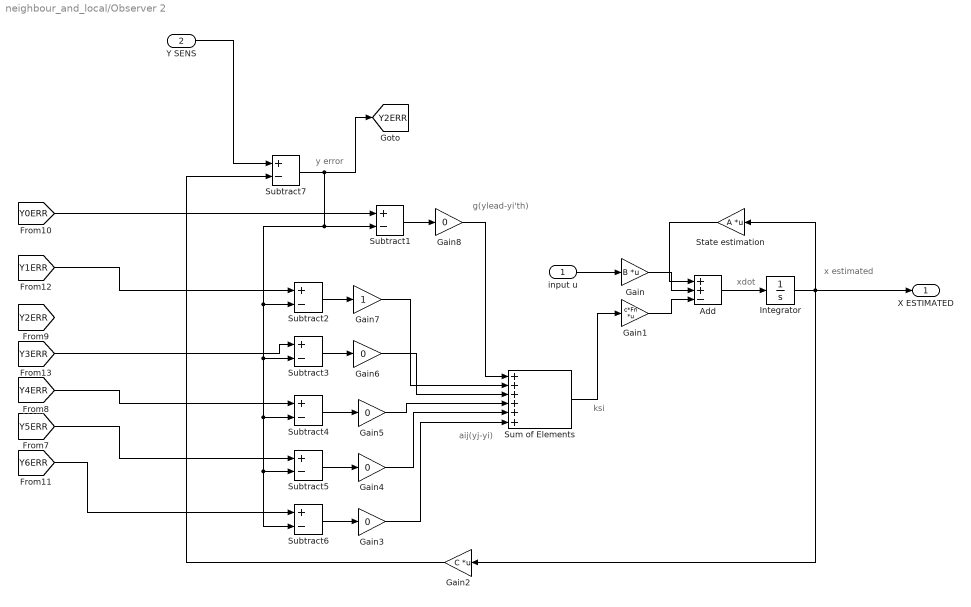
== system neighbour_and_local/Observer 2 ==
  note: aij(yj-yi)
  note: g(ylead-yi'th)
  note: ksi
  note: y error
  note: x estimated
  note: xdot
  input u : Inport
  Y SENS : Inport  Port=2
  Add : Sum  Inputs=++-
  Gain : Gain  Gain=B  Multiplication=Matrix(K*u)
  Gain1 : Gain  Gain=c*Fn  Multiplication=Matrix(K*u)
  Gain2 : Gain  Gain=C  Multiplication=Matrix(K*u)
  Gain{3..6,8} (5 alike) : Gain  Gain=0
  Gain7 : Gain
  Integrator : Integrator  InitialCondition=x0(:,2)
  State estimation : Gain  Gain=A  Multiplication=Matrix(K*u)
  Subtract{1..7} (7 alike) : Sum  Inputs=+-
  Sum of Elements : Sum  Inputs=++++++
  X ESTIMATED : Outport
  tag scope: Y2ERR=global
  wires:
  input u/1 -> Gain/1
  [Y0ERR] -> Subtract1/1
  Gain/1 -> Add/2
  Gain1/1 -> Add/3
  Add/1 -> Integrator/1
  State estimation/1 -> Add/1
  Integrator/1 -> X ESTIMATED/1, Gain2/1, State estimation/1
  Sum of Elements/1 -> Gain1/1
  Gain2/1 -> Subtract7/2
  [Y1ERR] -> Subtract2/1
  [Y3ERR] -> Subtract3/1
  [Y4ERR] -> Subtract4/1
  [Y5ERR] -> Subtract5/1
  [Y6ERR] -> Subtract6/1
  Subtract2/1 -> Gain7/1
  Subtract3/1 -> Gain6/1
  Subtract4/1 -> Gain5/1
  Subtract5/1 -> Gain4/1
  Subtract6/1 -> Gain3/1
  Subtract1/1 -> Gain8/1
  Gain8/1 -> Sum of Elements/1
  Gain7/1 -> Sum of Elements/2
  Gain6/1 -> Sum of Elements/3
  Gain3/1 -> Sum of Elements/6
  Gain5/1 -> Sum of Elements/4
  Gain4/1 -> Sum of Elements/5
  Subtract7/1 -> [Y2ERR], Subtract2/2, Subtract3/2, Subtract4/2, Subtract5/2, Subtract6/2, Subtract1/2
  Y SENS/1 -> Subtract7/1

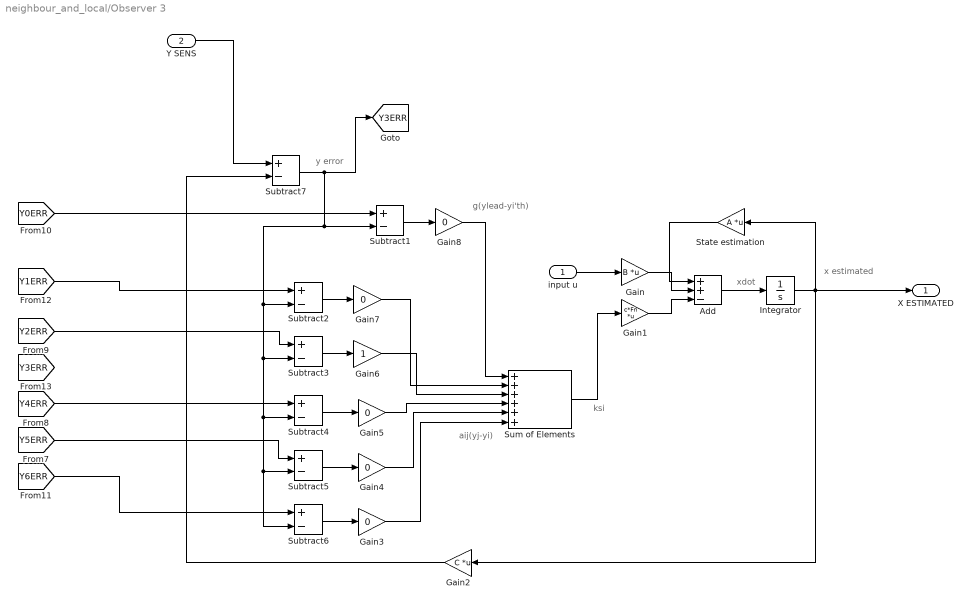
== system neighbour_and_local/Observer 3 ==
  note: aij(yj-yi)
  note: g(ylead-yi'th)
  note: ksi
  note: y error
  note: x estimated
  note: xdot
  input u : Inport
  Y SENS : Inport  Port=2
  Add : Sum  Inputs=++-
  Gain : Gain  Gain=B  Multiplication=Matrix(K*u)
  Gain1 : Gain  Gain=c*Fn  Multiplication=Matrix(K*u)
  Gain2 : Gain  Gain=C  Multiplication=Matrix(K*u)
  Gain{3..5,7..8} (5 alike) : Gain  Gain=0
  Gain6 : Gain
  Integrator : Integrator  InitialCondition=x0(:,3)
  State estimation : Gain  Gain=A  Multiplication=Matrix(K*u)
  Subtract{1..7} (7 alike) : Sum  Inputs=+-
  Sum of Elements : Sum  Inputs=++++++
  X ESTIMATED : Outport
  tag scope: Y3ERR=global
  wires:
  input u/1 -> Gain/1
  [Y0ERR] -> Subtract1/1
  Gain/1 -> Add/2
  Gain1/1 -> Add/3
  Add/1 -> Integrator/1
  State estimation/1 -> Add/1
  Integrator/1 -> X ESTIMATED/1, Gain2/1, State estimation/1
  Sum of Elements/1 -> Gain1/1
  Gain2/1 -> Subtract7/2
  [Y1ERR] -> Subtract2/1
  [Y2ERR] -> Subtract3/1
  [Y4ERR] -> Subtract4/1
  [Y5ERR] -> Subtract5/1
  [Y6ERR] -> Subtract6/1
  Subtract2/1 -> Gain7/1
  Subtract3/1 -> Gain6/1
  Subtract4/1 -> Gain5/1
  Subtract5/1 -> Gain4/1
  Subtract6/1 -> Gain3/1
  Subtract1/1 -> Gain8/1
  Gain8/1 -> Sum of Elements/1
  Gain7/1 -> Sum of Elements/2
  Gain6/1 -> Sum of Elements/3
  Gain3/1 -> Sum of Elements/6
  Gain5/1 -> Sum of Elements/4
  Gain4/1 -> Sum of Elements/5
  Subtract7/1 -> [Y3ERR], Subtract2/2, Subtract3/2, Subtract4/2, Subtract5/2, Subtract6/2, Subtract1/2
  Y SENS/1 -> Subtract7/1

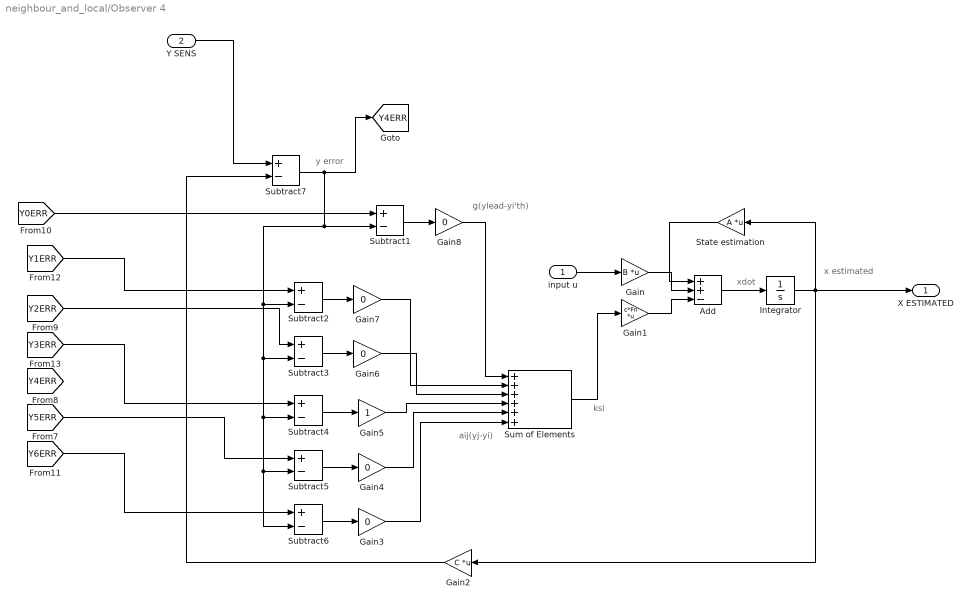
== system neighbour_and_local/Observer 4 ==
  note: aij(yj-yi)
  note: g(ylead-yi'th)
  note: ksi
  note: y error
  note: x estimated
  note: xdot
  input u : Inport
  Y SENS : Inport  Port=2
  Add : Sum  Inputs=++-
  Gain : Gain  Gain=B  Multiplication=Matrix(K*u)
  Gain1 : Gain  Gain=c*Fn  Multiplication=Matrix(K*u)
  Gain2 : Gain  Gain=C  Multiplication=Matrix(K*u)
  Gain{3..4,6..8} (5 alike) : Gain  Gain=0
  Gain5 : Gain
  Integrator : Integrator  InitialCondition=x0(:,4)
  State estimation : Gain  Gain=A  Multiplication=Matrix(K*u)
  Subtract{1..7} (7 alike) : Sum  Inputs=+-
  Sum of Elements : Sum  Inputs=++++++
  X ESTIMATED : Outport
  tag scope: Y4ERR=global
  wires:
  input u/1 -> Gain/1
  [Y0ERR] -> Subtract1/1
  Gain/1 -> Add/2
  Gain1/1 -> Add/3
  Add/1 -> Integrator/1
  State estimation/1 -> Add/1
  Integrator/1 -> X ESTIMATED/1, Gain2/1, State estimation/1
  Sum of Elements/1 -> Gain1/1
  Gain2/1 -> Subtract7/2
  [Y1ERR] -> Subtract2/1
  [Y2ERR] -> Subtract3/1
  [Y3ERR] -> Subtract4/1
  [Y5ERR] -> Subtract5/1
  [Y6ERR] -> Subtract6/1
  Subtract2/1 -> Gain7/1
  Subtract3/1 -> Gain6/1
  Subtract4/1 -> Gain5/1
  Subtract5/1 -> Gain4/1
  Subtract6/1 -> Gain3/1
  Subtract1/1 -> Gain8/1
  Gain8/1 -> Sum of Elements/1
  Gain7/1 -> Sum of Elements/2
  Gain6/1 -> Sum of Elements/3
  Gain3/1 -> Sum of Elements/6
  Gain5/1 -> Sum of Elements/4
  Gain4/1 -> Sum of Elements/5
  Subtract7/1 -> [Y4ERR], Subtract2/2, Subtract3/2, Subtract4/2, Subtract5/2, Subtract6/2, Subtract1/2
  Y SENS/1 -> Subtract7/1

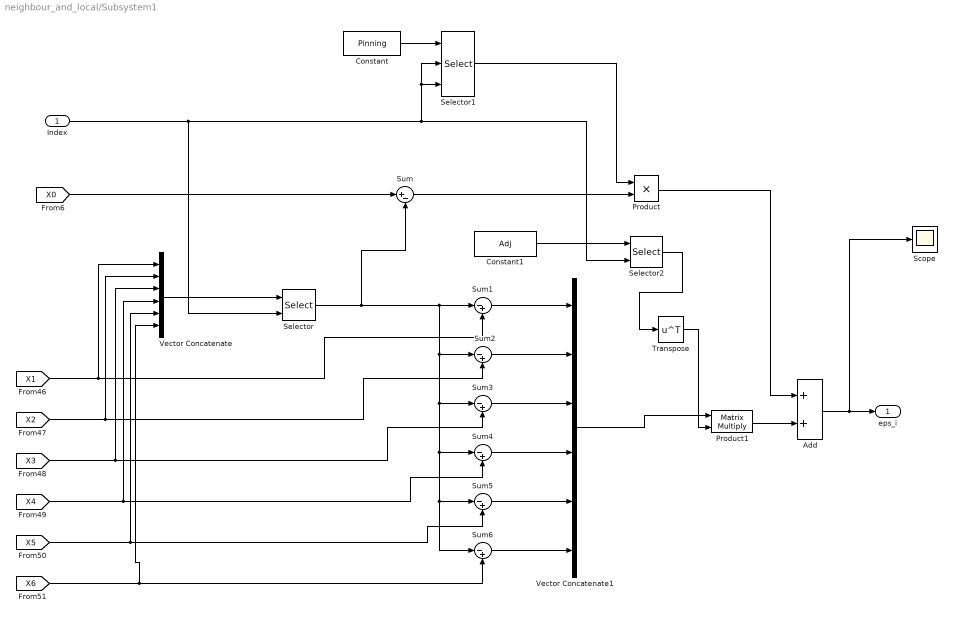
== system neighbour_and_local/Subsystem1 ==
  Index : Inport
  Add : Sum
  Constant : Constant  Value=Pinning
  Constant1 : Constant  Value=Adj
  Product : Product
  Product1 : Product  Multiplication=Matrix(*)
  Scope : Scope
  Selector : Selector  NumberOfDimensions=2  InputPortWidth=6  IndexOptions=Select all,Index vector (port)  Indices=[1 3],1  OutputSizes=1,1
  Selector1 : Selector  NumberOfDimensions=2  InputPortWidth=3  IndexOptions=Index vector (port),Index vector (port)  Indices=[1 3],1  OutputSizes=1,1
  Selector2 : Selector  NumberOfDimensions=2  InputPortWidth=3  IndexOptions=Index vector (port),Select all  Indices=[1 3],1  OutputSizes=1,1
  Sum : Sum  Inputs=|+-
  Sum{1..6} (6 alike) : Sum  Inputs=|-+
  Transpose : Math  Operator=transpose  SaturateOnIntegerOverflow=on
  Vector Concatenate : Concatenate  NumInputs=6  Mode=Multidimensional array  ConcatenateDimension=2
  Vector Concatenate1 : Concatenate  NumInputs=6  Mode=Multidimensional array  ConcatenateDimension=2
  eps_i : Outport
  wires:
  [X0] -> Sum/1
  Add/1 -> Scope/1, eps_i/1
  Index/1 -> Selector2/2, Selector1/3, Selector1/2, Selector/2
  Selector/1 -> Sum3/1, Sum6/1, Sum5/1, Sum4/1, Sum2/1, Sum1/1, Sum/2
  Constant/1 -> Selector1/1
  Sum/1 -> Product/2
  Selector1/1 -> Product/1
  Product/1 -> Add/1
  Constant1/1 -> Selector2/1
  Sum1/1 -> Vector Concatenate1/1
  Sum2/1 -> Vector Concatenate1/2
  Sum3/1 -> Vector Concatenate1/3
  Sum4/1 -> Vector Concatenate1/4
  Sum5/1 -> Vector Concatenate1/5
  Sum6/1 -> Vector Concatenate1/6
  Vector Concatenate1/1 -> Product1/1
  Product1/1 -> Add/2
  [X1] -> Vector Concatenate/1, Sum1/2
  [X2] -> Vector Concatenate/2, Sum2/2
  [X3] -> Vector Concatenate/3, Sum3/2
  [X4] -> Vector Concatenate/4, Sum4/2
  [X5] -> Vector Concatenate/5, Sum5/2
  [X6] -> Vector Concatenate/6, Sum6/2
  Vector Concatenate/1 -> Selector/1
  Selector2/1 -> Transpose/1
  Transpose/1 -> Product1/2

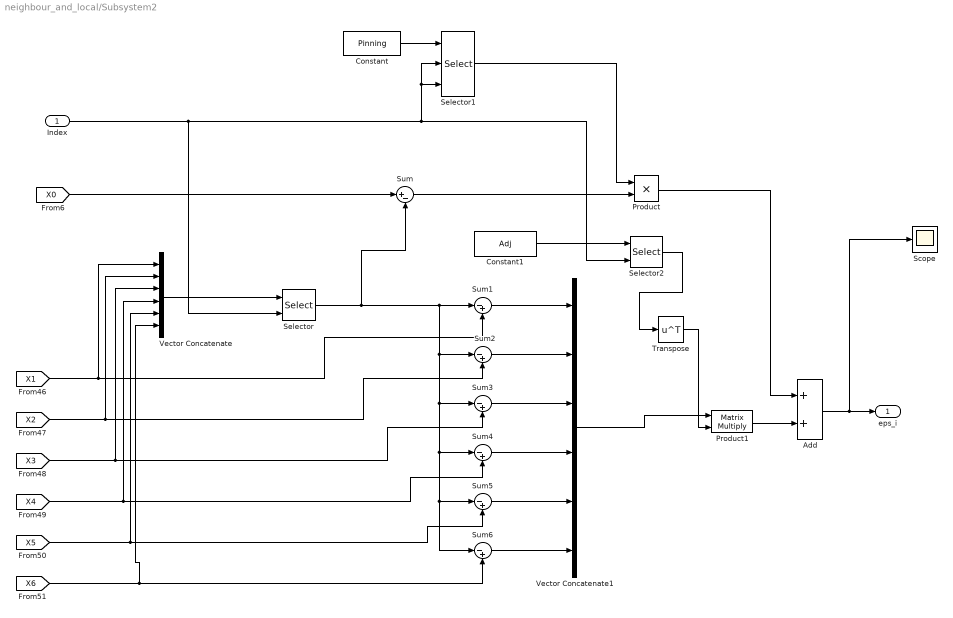
== system neighbour_and_local/Subsystem2 ==
  Index : Inport
  Add : Sum
  Constant : Constant  Value=Pinning
  Constant1 : Constant  Value=Adj
  Product : Product
  Product1 : Product  Multiplication=Matrix(*)
  Scope : Scope
  Selector : Selector  NumberOfDimensions=2  InputPortWidth=6  IndexOptions=Select all,Index vector (port)  Indices=[1 3],1  OutputSizes=1,1
  Selector1 : Selector  NumberOfDimensions=2  InputPortWidth=3  IndexOptions=Index vector (port),Index vector (port)  Indices=[1 3],1  OutputSizes=1,1
  Selector2 : Selector  NumberOfDimensions=2  InputPortWidth=3  IndexOptions=Index vector (port),Select all  Indices=[1 3],1  OutputSizes=1,1
  Sum : Sum  Inputs=|+-
  Sum{1..6} (6 alike) : Sum  Inputs=|-+
  Transpose : Math  Operator=transpose  SaturateOnIntegerOverflow=on
  Vector Concatenate : Concatenate  NumInputs=6  Mode=Multidimensional array  ConcatenateDimension=2
  Vector Concatenate1 : Concatenate  NumInputs=6  Mode=Multidimensional array  ConcatenateDimension=2
  eps_i : Outport
  wires:
  [X0] -> Sum/1
  Add/1 -> Scope/1, eps_i/1
  Index/1 -> Selector2/2, Selector1/3, Selector1/2, Selector/2
  Selector/1 -> Sum3/1, Sum6/1, Sum5/1, Sum4/1, Sum2/1, Sum1/1, Sum/2
  Constant/1 -> Selector1/1
  Sum/1 -> Product/2
  Selector1/1 -> Product/1
  Product/1 -> Add/1
  Constant1/1 -> Selector2/1
  Sum1/1 -> Vector Concatenate1/1
  Sum2/1 -> Vector Concatenate1/2
  Sum3/1 -> Vector Concatenate1/3
  Sum4/1 -> Vector Concatenate1/4
  Sum5/1 -> Vector Concatenate1/5
  Sum6/1 -> Vector Concatenate1/6
  Vector Concatenate1/1 -> Product1/1
  Product1/1 -> Add/2
  [X1] -> Vector Concatenate/1, Sum1/2
  [X2] -> Vector Concatenate/2, Sum2/2
  [X3] -> Vector Concatenate/3, Sum3/2
  [X4] -> Vector Concatenate/4, Sum4/2
  [X5] -> Vector Concatenate/5, Sum5/2
  [X6] -> Vector Concatenate/6, Sum6/2
  Vector Concatenate/1 -> Selector/1
  Selector2/1 -> Transpose/1
  Transpose/1 -> Product1/2

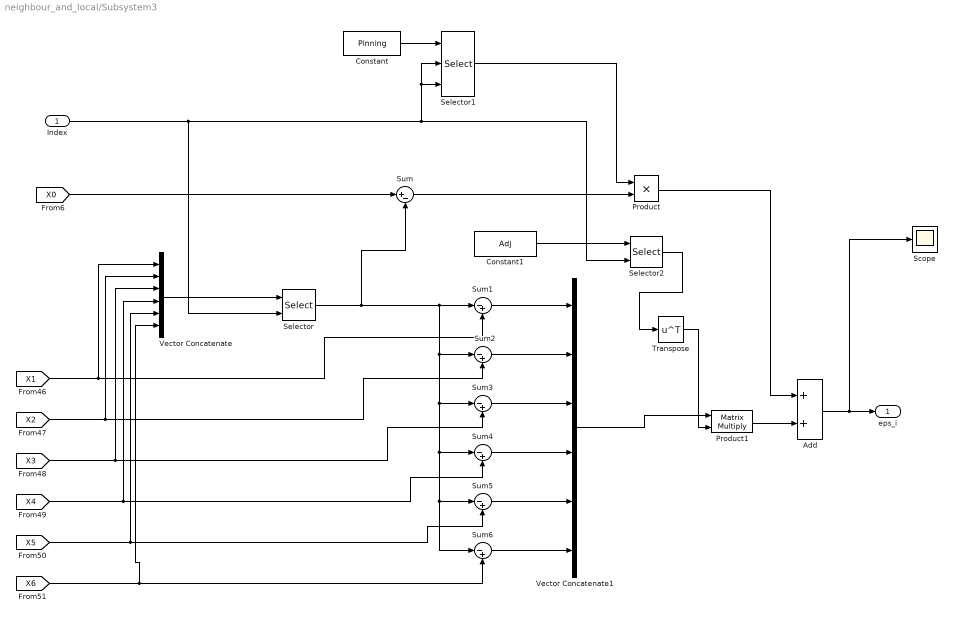
== system neighbour_and_local/Subsystem3 ==
  Index : Inport
  Add : Sum
  Constant : Constant  Value=Pinning
  Constant1 : Constant  Value=Adj
  Product : Product
  Product1 : Product  Multiplication=Matrix(*)
  Scope : Scope
  Selector : Selector  NumberOfDimensions=2  InputPortWidth=6  IndexOptions=Select all,Index vector (port)  Indices=[1 3],1  OutputSizes=1,1
  Selector1 : Selector  NumberOfDimensions=2  InputPortWidth=3  IndexOptions=Index vector (port),Index vector (port)  Indices=[1 3],1  OutputSizes=1,1
  Selector2 : Selector  NumberOfDimensions=2  InputPortWidth=3  IndexOptions=Index vector (port),Select all  Indices=[1 3],1  OutputSizes=1,1
  Sum : Sum  Inputs=|+-
  Sum{1..6} (6 alike) : Sum  Inputs=|-+
  Transpose : Math  Operator=transpose  SaturateOnIntegerOverflow=on
  Vector Concatenate : Concatenate  NumInputs=6  Mode=Multidimensional array  ConcatenateDimension=2
  Vector Concatenate1 : Concatenate  NumInputs=6  Mode=Multidimensional array  ConcatenateDimension=2
  eps_i : Outport
  wires:
  [X0] -> Sum/1
  Add/1 -> Scope/1, eps_i/1
  Index/1 -> Selector2/2, Selector1/3, Selector1/2, Selector/2
  Selector/1 -> Sum3/1, Sum6/1, Sum5/1, Sum4/1, Sum2/1, Sum1/1, Sum/2
  Constant/1 -> Selector1/1
  Sum/1 -> Product/2
  Selector1/1 -> Product/1
  Product/1 -> Add/1
  Constant1/1 -> Selector2/1
  Sum1/1 -> Vector Concatenate1/1
  Sum2/1 -> Vector Concatenate1/2
  Sum3/1 -> Vector Concatenate1/3
  Sum4/1 -> Vector Concatenate1/4
  Sum5/1 -> Vector Concatenate1/5
  Sum6/1 -> Vector Concatenate1/6
  Vector Concatenate1/1 -> Product1/1
  Product1/1 -> Add/2
  [X1] -> Vector Concatenate/1, Sum1/2
  [X2] -> Vector Concatenate/2, Sum2/2
  [X3] -> Vector Concatenate/3, Sum3/2
  [X4] -> Vector Concatenate/4, Sum4/2
  [X5] -> Vector Concatenate/5, Sum5/2
  [X6] -> Vector Concatenate/6, Sum6/2
  Vector Concatenate/1 -> Selector/1
  Selector2/1 -> Transpose/1
  Transpose/1 -> Product1/2

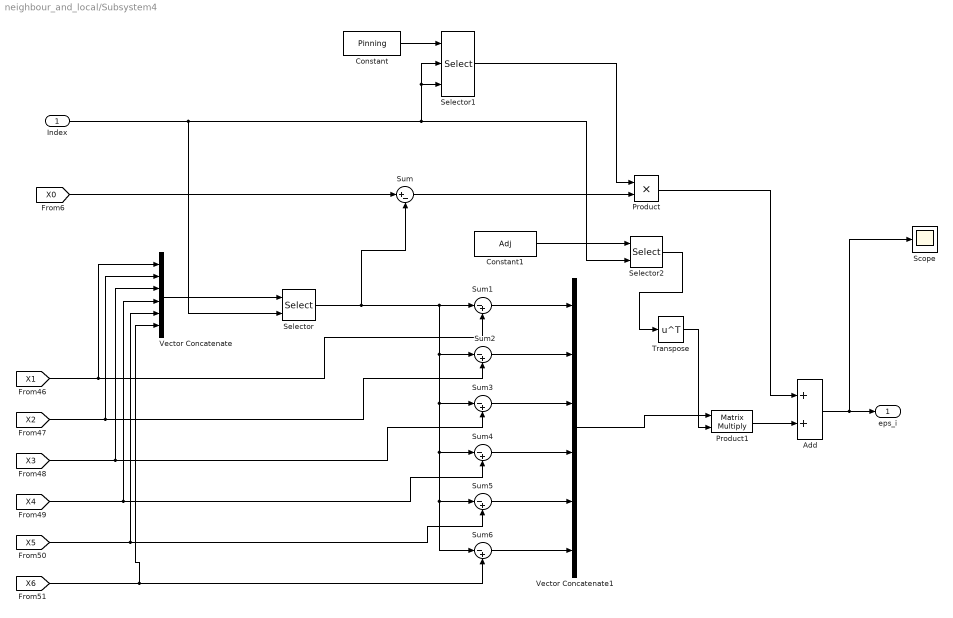
== system neighbour_and_local/Subsystem4 ==
  Index : Inport
  Add : Sum
  Constant : Constant  Value=Pinning
  Constant1 : Constant  Value=Adj
  Product : Product
  Product1 : Product  Multiplication=Matrix(*)
  Scope : Scope
  Selector : Selector  NumberOfDimensions=2  InputPortWidth=6  IndexOptions=Select all,Index vector (port)  Indices=[1 3],1  OutputSizes=1,1
  Selector1 : Selector  NumberOfDimensions=2  InputPortWidth=3  IndexOptions=Index vector (port),Index vector (port)  Indices=[1 3],1  OutputSizes=1,1
  Selector2 : Selector  NumberOfDimensions=2  InputPortWidth=3  IndexOptions=Index vector (port),Select all  Indices=[1 3],1  OutputSizes=1,1
  Sum : Sum  Inputs=|+-
  Sum{1..6} (6 alike) : Sum  Inputs=|-+
  Transpose : Math  Operator=transpose  SaturateOnIntegerOverflow=on
  Vector Concatenate : Concatenate  NumInputs=6  Mode=Multidimensional array  ConcatenateDimension=2
  Vector Concatenate1 : Concatenate  NumInputs=6  Mode=Multidimensional array  ConcatenateDimension=2
  eps_i : Outport
  wires:
  [X0] -> Sum/1
  Add/1 -> Scope/1, eps_i/1
  Index/1 -> Selector2/2, Selector1/3, Selector1/2, Selector/2
  Selector/1 -> Sum3/1, Sum6/1, Sum5/1, Sum4/1, Sum2/1, Sum1/1, Sum/2
  Constant/1 -> Selector1/1
  Sum/1 -> Product/2
  Selector1/1 -> Product/1
  Product/1 -> Add/1
  Constant1/1 -> Selector2/1
  Sum1/1 -> Vector Concatenate1/1
  Sum2/1 -> Vector Concatenate1/2
  Sum3/1 -> Vector Concatenate1/3
  Sum4/1 -> Vector Concatenate1/4
  Sum5/1 -> Vector Concatenate1/5
  Sum6/1 -> Vector Concatenate1/6
  Vector Concatenate1/1 -> Product1/1
  Product1/1 -> Add/2
  [X1] -> Vector Concatenate/1, Sum1/2
  [X2] -> Vector Concatenate/2, Sum2/2
  [X3] -> Vector Concatenate/3, Sum3/2
  [X4] -> Vector Concatenate/4, Sum4/2
  [X5] -> Vector Concatenate/5, Sum5/2
  [X6] -> Vector Concatenate/6, Sum6/2
  Vector Concatenate/1 -> Selector/1
  Selector2/1 -> Transpose/1
  Transpose/1 -> Product1/2

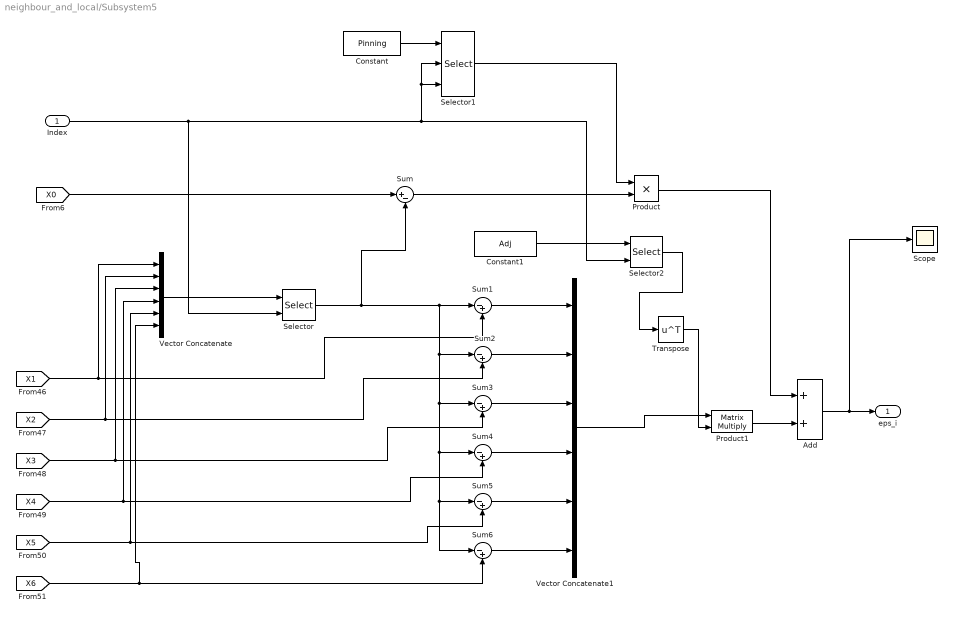
== system neighbour_and_local/Subsystem5 ==
  Index : Inport
  Add : Sum
  Constant : Constant  Value=Pinning
  Constant1 : Constant  Value=Adj
  Product : Product
  Product1 : Product  Multiplication=Matrix(*)
  Scope : Scope
  Selector : Selector  NumberOfDimensions=2  InputPortWidth=6  IndexOptions=Select all,Index vector (port)  Indices=[1 3],1  OutputSizes=1,1
  Selector1 : Selector  NumberOfDimensions=2  InputPortWidth=3  IndexOptions=Index vector (port),Index vector (port)  Indices=[1 3],1  OutputSizes=1,1
  Selector2 : Selector  NumberOfDimensions=2  InputPortWidth=3  IndexOptions=Index vector (port),Select all  Indices=[1 3],1  OutputSizes=1,1
  Sum : Sum  Inputs=|+-
  Sum{1..6} (6 alike) : Sum  Inputs=|-+
  Transpose : Math  Operator=transpose  SaturateOnIntegerOverflow=on
  Vector Concatenate : Concatenate  NumInputs=6  Mode=Multidimensional array  ConcatenateDimension=2
  Vector Concatenate1 : Concatenate  NumInputs=6  Mode=Multidimensional array  ConcatenateDimension=2
  eps_i : Outport
  wires:
  [X0] -> Sum/1
  Add/1 -> Scope/1, eps_i/1
  Index/1 -> Selector2/2, Selector1/3, Selector1/2, Selector/2
  Selector/1 -> Sum3/1, Sum6/1, Sum5/1, Sum4/1, Sum2/1, Sum1/1, Sum/2
  Constant/1 -> Selector1/1
  Sum/1 -> Product/2
  Selector1/1 -> Product/1
  Product/1 -> Add/1
  Constant1/1 -> Selector2/1
  Sum1/1 -> Vector Concatenate1/1
  Sum2/1 -> Vector Concatenate1/2
  Sum3/1 -> Vector Concatenate1/3
  Sum4/1 -> Vector Concatenate1/4
  Sum5/1 -> Vector Concatenate1/5
  Sum6/1 -> Vector Concatenate1/6
  Vector Concatenate1/1 -> Product1/1
  Product1/1 -> Add/2
  [X1] -> Vector Concatenate/1, Sum1/2
  [X2] -> Vector Concatenate/2, Sum2/2
  [X3] -> Vector Concatenate/3, Sum3/2
  [X4] -> Vector Concatenate/4, Sum4/2
  [X5] -> Vector Concatenate/5, Sum5/2
  [X6] -> Vector Concatenate/6, Sum6/2
  Vector Concatenate/1 -> Selector/1
  Selector2/1 -> Transpose/1
  Transpose/1 -> Product1/2

== system neighbour_and_local/Subsystem6 ==
  Index : Inport
  Add : Sum
  Constant : Constant  Value=Pinning
  Constant1 : Constant  Value=Adj
  Product : Product
  Product1 : Product  Multiplication=Matrix(*)
  Scope : Scope
  Selector : Selector  NumberOfDimensions=2  InputPortWidth=6  IndexOptions=Select all,Index vector (port)  Indices=[1 3],1  OutputSizes=1,1
  Selector1 : Selector  NumberOfDimensions=2  InputPortWidth=3  IndexOptions=Index vector (port),Index vector (port)  Indices=[1 3],1  OutputSizes=1,1
  Selector2 : Selector  NumberOfDimensions=2  InputPortWidth=3  IndexOptions=Index vector (port),Select all  Indices=[1 3],1  OutputSizes=1,1
  Sum : Sum  Inputs=|+-
  Sum{1..6} (6 alike) : Sum  Inputs=|-+
  Transpose : Math  Operator=transpose  SaturateOnIntegerOverflow=on
  Vector Concatenate : Concatenate  NumInputs=6  Mode=Multidimensional array  ConcatenateDimension=2
  Vector Concatenate1 : Concatenate  NumInputs=6  Mode=Multidimensional array  ConcatenateDimension=2
  eps_i : Outport
  wires:
  [X0] -> Sum/1
  Add/1 -> Scope/1, eps_i/1
  Index/1 -> Selector2/2, Selector1/3, Selector1/2, Selector/2
  Selector/1 -> Sum3/1, Sum6/1, Sum5/1, Sum4/1, Sum2/1, Sum1/1, Sum/2
  Constant/1 -> Selector1/1
  Sum/1 -> Product/2
  Selector1/1 -> Product/1
  Product/1 -> Add/1
  Constant1/1 -> Selector2/1
  Sum1/1 -> Vector Concatenate1/1
  Sum2/1 -> Vector Concatenate1/2
  Sum3/1 -> Vector Concatenate1/3
  Sum4/1 -> Vector Concatenate1/4
  Sum5/1 -> Vector Concatenate1/5
  Sum6/1 -> Vector Concatenate1/6
  Vector Concatenate1/1 -> Product1/1
  Product1/1 -> Add/2
  [X1] -> Vector Concatenate/1, Sum1/2
  [X2] -> Vector Concatenate/2, Sum2/2
  [X3] -> Vector Concatenate/3, Sum3/2
  [X4] -> Vector Concatenate/4, Sum4/2
  [X5] -> Vector Concatenate/5, Sum5/2
  [X6] -> Vector Concatenate/6, Sum6/2
  Vector Concatenate/1 -> Selector/1
  Selector2/1 -> Transpose/1
  Transpose/1 -> Product1/2
